simulink subsystem "RoboCar_test_4"  (R2023a)
settings: Solver=VariableStepAuto  StartTime=0.0  StopTime=10.0  RelTol=1e-3
settings Model: Creator=Franz  LastModifiedBy=Franz

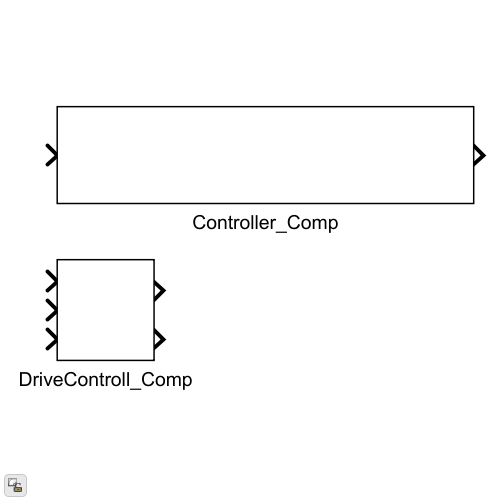
[thumbnail: Simulink's stored preview of the top-level diagram]
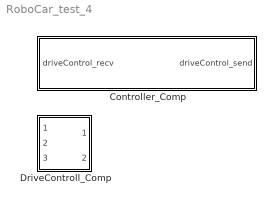
== system RoboCar_test_4 ==
  Controller_Comp : Subsystem
  DriveControll_Comp : Subsystem

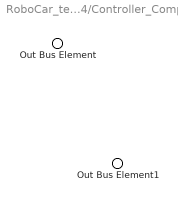
== system RoboCar_test_4/Controller_Comp ==
  Out Bus Element : Inport  PortName=driveControl_recv  Element=signal1
  Out Bus Element1 : Outport  PortName=driveControl_send  Element=signal1

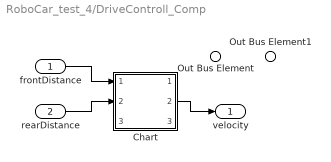
== system RoboCar_test_4/DriveControll_Comp ==
  frontDistance : Inport
  rearDistance : Inport  Port=2
  Out Bus Element : Inport  Port=3  PortName=driveControl_recv  Element=signal1
  Chart : Stateflow chart  TreatAsAtomicUnit=on
  velocity : Outport
  Out Bus Element1 : Outport  Port=2  PortName=driveControl_send  Element=signal1
  wires:
  rearDistance/1 -> Chart/2(rearDistance)
  frontDistance/1 -> Chart/1(frontDistance)
  Chart/2(velocity) -> velocity/1

== stateflow chart RoboCar_test_4/DriveControll_Comp/Chart ==
  state chart
    state chartRegion [parallel]
      settings: executionOrder=1
      state DriveControlComponent
        state driveControlPort [parallel]
          settings: executionOrder=1
          state Idle
          state WaitforCoordinator
          state WaitForOvertaking
          (default) -> Idle
          WaitForOvertaking -> Idle : [communicator_recv == 2]{velocity = 50;}
          WaitforCoordinator -> WaitForOvertaking [order 2] : grantPermission{communicator_send = 1;}
          WaitforCoordinator -> Idle [order 1] : denyPermission{driveControl_send = 4;}
          Idle -> WaitforCoordinator : [frontDistance <100 && rearDistance > 1]{send(OvertakingRequested), coordination_Successfull = true;}
        state driving [parallel]
          settings: executionOrder=2
      (default) -> DriveControlComponent
  (default) -> chart
  data: frontDistance input Int32; rearDistance input; driveControl_send output; velocity output; coordination_Successfull local; communicator_recv input; communicator_send output
  events: denyPermission local FUNCTION_CALL_EVENT; grantPermission local FUNCTION_CALL_EVENT; OvertakingRequested local FUNCTION_CALL_EVENT
